simulink model "Main_C0_C3"  (R2023a)
settings: Solver=ode15s  StartTime=0.0  StopTime=1  RelTol=1e-3
model workspace (MAT data in the model file):
  C_IVD = 0.05
  E_IVD1 = 2.1
  E_IVD2 = 2.2
  E_IVD3 = 1.1
  E_IVD4 = 1.7
  E_IVD5 = 3.2
  IVD1 : object (value not decoded)
  IVD2 : object (value not decoded)
  IVD3 : object (value not decoded)
  IVD4 : object (value not decoded)
  IVD5 : object (value not decoded)
  eo_color = [1 0 0]
  io_color = [0 1 0]
  longissimus_color = [1 0 1]
  multifidus_color = [0 1 1]
  muscle_radius = 1
  psoas_color = [0 0 1]
  ra_color = [1 1 0.5]
symbols that are objects in the model workspace (value not decoded): IVD1, IVD2, IVD3, IVD4, IVD5
undefined symbols (not defined in the file or in its folder): AbdFlex, E_TLFflex, IAP_activation_AbdFlex, IAP_Pa, LeftAbdominalMuscleForce, LeftBackMuscleForce, LeftTransverse1MuscleForce, LeftTransverse2MuscleForce, RightAbdominalMuscleForce, RightBackMuscleForce, RightTransverse1MuscleForce, RightTransverse2MuscleForce, TLFflex2, X, Y, Z
libraries: nesl_utility x1235, sm_lib x960, fl_lib x6, simulink_extras x2
(part 5 of 37)

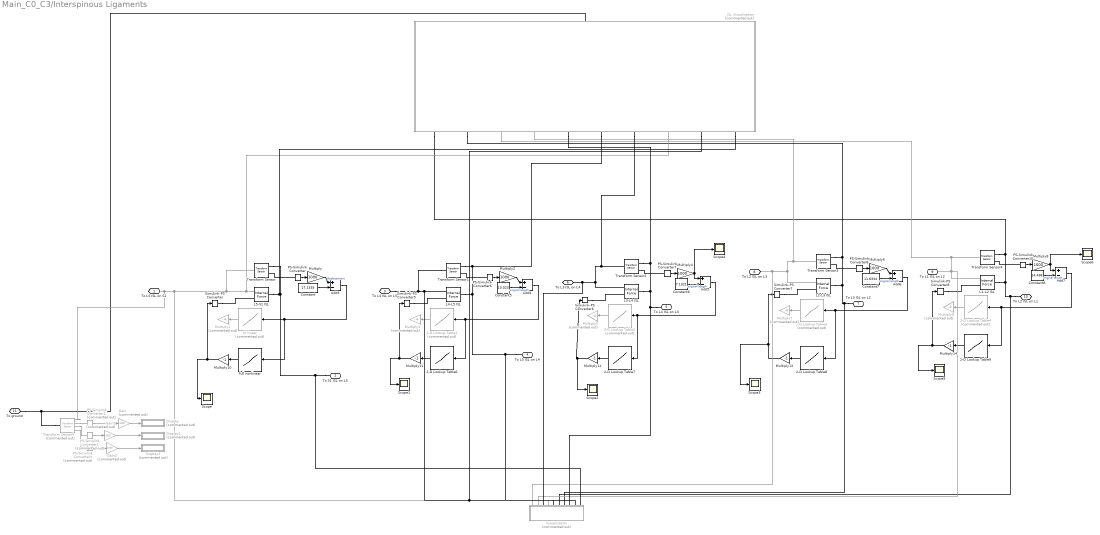
== system Main_C0_C3/Interspinous Ligaments ==
  2-D Lookup Table1 : Lookup_n-D  Commented=on  NumberOfTableDimensions=1  BreakpointsForDimension1=[0;0.1802;1.802;3.604;10.812]  BreakpointsForDimension2=[1:3]  Table=[0;0;4.82625;10.53;48.2625]  InternalRulePriority=Speed  RndMeth=Simplest
  2-D Lookup Table2 : Lookup_n-D  Commented=on  NumberOfTableDimensions=1  BreakpointsForDimension1=[0;0.054;0.54;1.08;3.24]  BreakpointsForDimension2=[1:3]  Table=[0;0;4.82625;10.53;48.2625]  InternalRulePriority=Speed  RndMeth=Simplest
  2-D Lookup Table3 : Lookup_n-D  Commented=on  NumberOfTableDimensions=1  BreakpointsForDimension1=[0;0.071;0.71;1.42;4.26]  BreakpointsForDimension2=[1:3]  Table=[0;0;4.82625;10.53;48.2625]  InternalRulePriority=Speed  RndMeth=Simplest
  2-D Lookup Table4 : Lookup_n-D  Commented=on  NumberOfTableDimensions=1  BreakpointsForDimension1=[0;0.105;1.05;2.1;6.3]  BreakpointsForDimension2=[1:3]  Table=[0;0;4.82625;10.53;48.2625]  InternalRulePriority=Speed  RndMeth=Simplest
  2-D Lookup Table6 : Lookup_n-D  NumberOfTableDimensions=1  BreakpointsForDimension1=[0;0.788999;0.899258;1.033633;1.693478;1.826126;1.958782;3.004578;3.254415;3.518032;5.870167;6.506087;7.157553]  BreakpointsForDimension2=[1:3]  Table=[0;12.24469;14.30802;16.68834;29.86456;31.92651;34.46617;57.49141;64.0048;70.67658;144.8958;168.9015;195.6133]  InternalRulePriority=Speed  RndMeth=Simplest
  2-D Lookup Table7 : Lookup_n-D  NumberOfTableDimensions=1  BreakpointsForDimension1=[0;0.432098;0.492482;0.566074;0.92744;1.000085;1.072735;1.645469;1.782294;1.926665;3.214821;3.563086;3.919864]  BreakpointsForDimension2=[1:3]  Table=[0;12.24469;14.30802;16.68834;29.86456;31.92651;34.46617;57.49141;64.0048;70.67658;144.8958;168.9015;195.6133]  InternalRulePriority=Speed  RndMeth=Simplest
  2-D Lookup Table8 : Lookup_n-D  NumberOfTableDimensions=1  BreakpointsForDimension1=[0;0.70481;0.803304;0.923341;1.512778;1.631272;1.749773;2.683979;2.907157;3.142646;5.2438;5.811865;6.393817]  BreakpointsForDimension2=[1:3]  Table=[0;12.24469;14.30802;16.68834;29.86456;31.92651;34.46617;57.49141;64.0048;70.67658;144.8958;168.9015;195.6133]  InternalRulePriority=Speed  RndMeth=Simplest
  2-D Lookup Table9 : Lookup_n-D  NumberOfTableDimensions=1  BreakpointsForDimension1=[0;0.581192;0.662411;0.761395;1.247449;1.34516;1.442878;2.213232;2.397266;2.591452;4.324082;4.792513;5.272396]  BreakpointsForDimension2=[1:3]  Table=[0;12.24469;14.30802;16.68834;29.86456;31.92651;34.46617;57.49141;64.0048;70.67658;144.8958;168.9015;195.6133]  InternalRulePriority=Speed  RndMeth=Simplest
  Add{3..7} (5 alike) : Sum  Inputs=+-
  Constant : Constant  Value=17.1335
  Constant5 : Constant  Value=13.023
  Constant6 : Constant  Value=7.1321
  Constant7 : Constant  Value=11.6334
  Constant8 : Constant  Value=14.438
  Display : Display  Commented=on
  Display1 : Display  Commented=on
  Display2 : Display  Commented=on
  Gain : Gain  Commented=on  Gain=1000
  Gain1 : Gain  Commented=on  Gain=1000
  Gain2 : Gain  Commented=on  Gain=1000
  ISL Visualization : Subsystem  Commented=on
  L1-L2 ISL : sm_lib/Forces and Torques/Internal Force
  L2-L3 ISL : sm_lib/Forces and Torques/Internal Force
  L3-L4 ISL : sm_lib/Forces and Torques/Internal Force
  L4-L5 ISL : sm_lib/Forces and Torques/Internal Force
  L5-S1 ISL : sm_lib/Forces and Torques/Internal Force
  Multiply{,2,4,6,8} (5 alike) : Gain  Gain=1000
  Multiply{1,3,5,7,9} (5 alike) : Gain  Commented=on  Gain=-4
  Multiply{10..14} (5 alike) : Gain  Gain=-1
  PS-Simulink Converter{,6..8,10} (5 alike) : nesl_utility/PS-Simulink Converter  PhysicalDomain=network_engine_domain  SubClassName=ps_output  LeftPortType=input  RightPortType=output  PseudoPeriodic=off  Frequencies=[]  VectorFormat=inherit  Unit=inherit  AffineConversion=off
  PS-Simulink Converter1 : nesl_utility/PS-Simulink Converter  Commented=on  PhysicalDomain=network_engine_domain  SubClassName=ps_output  LeftPortType=input  RightPortType=output  PseudoPeriodic=off  Frequencies=[]  VectorFormat=inherit  Unit=inherit  AffineConversion=off
  PS-Simulink Converter2 : nesl_utility/PS-Simulink Converter  Commented=on  PhysicalDomain=network_engine_domain  SubClassName=ps_output  LeftPortType=input  RightPortType=output  PseudoPeriodic=off  Frequencies=[]  VectorFormat=inherit  Unit=inherit  AffineConversion=off
  PS-Simulink Converter3 : nesl_utility/PS-Simulink Converter  Commented=on  PhysicalDomain=network_engine_domain  SubClassName=ps_output  LeftPortType=input  RightPortType=output  PseudoPeriodic=off  Frequencies=[]  VectorFormat=inherit  Unit=inherit  AffineConversion=off
  Scope{,1..6} (7 alike) : Scope
  Simulink-PS Converter{,5..8} (5 alike) : nesl_utility/Simulink-PS Converter  PhysicalDomain=network_engine_domain  SubClassName=ps_input  LeftPortType=input  RightPortType=output  PseudoPeriodic=off  Frequencies=[]  NoiseDistribution=none  NoiseParameters=[]  Unit=1  AffineConversion=off  FilteringAndDerivatives=provide  SimscapeFilterOrder=1  InputFilterTimeConstant=0.001  UdotUserProvided=0
  Transform Sensor{,1..4} (5 alike) : sm_lib/Frames and Transforms/Transform Sensor  MeasurementFrame=World  RotationSequence=XYX  SenseAngle=off  SenseAxis=off  SenseQ=off  SenseR=off  SenseRotationSequence=off  SenseOmegaX=off  SenseOmegaY=off  SenseOmegaZ=off  SenseQDot=off  SenseRDot=off  SenseRotationSequenceDot=off  SenseAlphaX=off  SenseAlphaY=off  SenseAlphaZ=off  SenseQDDot=off  SenseRDDot=off  SenseX=off  SenseY=off  SenseZ=off  SenseRad=off  SenseAzim=off  SenseDist=on  SenseInc=off  SenseXDot=off  SenseYDot=off  SenseZDot=off  SenseRadDot=off  SenseAzimDot=off  SenseDistDot=off  SenseIncDot=off  SenseXDDot=off  SenseYDDot=off  SenseZDDot=off  SenseRadDDot=off  SenseAzimDDot=off  SenseDistDDot=off  SenseIncDDot=off
  Transform Sensor5 : sm_lib/Frames and Transforms/Transform Sensor  Commented=on  MeasurementFrame=World  RotationSequence=XYZ  SenseAngle=off  SenseAxis=off  SenseQ=off  SenseR=off  SenseRotationSequence=off  SenseOmegaX=off  SenseOmegaY=off  SenseOmegaZ=off  SenseQDot=off  SenseRDot=off  SenseRotationSequenceDot=off  SenseAlphaX=off  SenseAlphaY=off  SenseAlphaZ=off  SenseQDDot=off  SenseRDDot=off  SenseX=on  SenseY=on  SenseZ=on  SenseRad=off  SenseAzim=off  SenseDist=off  SenseInc=off  SenseXDot=off  SenseYDot=off  SenseZDot=off  SenseRadDot=off  SenseAzimDot=off  SenseDistDot=off  SenseIncDot=off  SenseXDDot=off  SenseYDDot=off  SenseZDDot=off  SenseRadDDot=off  SenseAzimDDot=off  SenseDistDDot=off  SenseIncDDot=off
  Visualization : Subsystem  Commented=on
  bi linear : Lookup_n-D  Commented=on  NumberOfTableDimensions=1  BreakpointsForDimension1=[0;0.1802;1.802;3.604;10.812]  BreakpointsForDimension2=[1:3]  Table=[0;0;4.82625;10.53;48.2625]  InternalRulePriority=Speed  RndMeth=Simplest
  full nonlinear : Lookup_n-D  NumberOfTableDimensions=1  BreakpointsForDimension1=[0;1.038033;1.183094;1.359883;2.227997;2.402513;2.57704;3.952924;4.281618;4.628442;7.722991;8.559628;9.41672]  BreakpointsForDimension2=[1:3]  Table=[0;12.24469;14.30802;16.68834;29.86456;31.92651;34.46617;57.49141;64.0048;70.67658;144.8958;168.9015;195.6133]  InternalRulePriority=Speed  RndMeth=Simplest
  To L5 ISL on S1 : PMIOPort  Side=Left
  To S1 ISL on L5 : PMIOPort  Port=2  Side=Left
  To L4 ISL on L5 : PMIOPort  Port=3  Side=Left
  To L5 ISL on L4 : PMIOPort  Port=4  Side=Left
  To L4 ISL on L3 : PMIOPort  Port=5  Side=Left
  To L3 ISL on L4 : PMIOPort  Port=6  Side=Left
  To L3 ISL on L2 : PMIOPort  Port=7  Side=Left
  To L2 ISL on L3 : PMIOPort  Port=8  Side=Left
  To L1 ISL on L2 : PMIOPort  Port=9  Side=Left
  To L2 ISL on L1 : PMIOPort  Port=10  Side=Left
  "To ground " : PMIOPort  Port=11  Side=Left
  wires:
  Multiply10/1 -> Simulink-PS Converter/1, Scope/1
  Gain/1 -> Display/1
  Gain1/1 -> Display1/1
  Gain2/1 -> Display2/1
  PS-Simulink Converter3/1 -> Gain2/1
  PS-Simulink Converter2/1 -> Gain1/1
  PS-Simulink Converter1/1 -> Gain/1
  Multiply14/1 -> Scope5/1, Simulink-PS Converter8/1
  Multiply13/1 -> Simulink-PS Converter7/1, Scope3/1
  Multiply12/1 -> Simulink-PS Converter6/1, Scope2/1
  Multiply11/1 -> Simulink-PS Converter5/1, Scope1/1
  2-D Lookup Table9/1 -> Multiply14/1
  2-D Lookup Table8/1 -> Multiply13/1
  2-D Lookup Table7/1 -> Multiply12/1
  2-D Lookup Table6/1 -> Multiply11/1
  full nonlinear/1 -> Multiply10/1
  Add7/1 -> 2-D Lookup Table4/1, 2-D Lookup Table9/1
  Constant8/1 -> Add7/2  "original length"
  Constant7/1 -> Add6/2  "original length"
  Add6/1 -> 2-D Lookup Table3/1, 2-D Lookup Table8/1
  Add5/1 -> 2-D Lookup Table2/1, 2-D Lookup Table7/1
  Constant6/1 -> Add5/2  "original length"
  Constant5/1 -> Add4/2  "original length"
  Add4/1 -> 2-D Lookup Table1/1, 2-D Lookup Table6/1
  Multiply/1 -> Add3/1  "displacement"
  PS-Simulink Converter10/1 -> Multiply8/1
  PS-Simulink Converter8/1 -> Multiply6/1
  Multiply6/1 -> Add6/1
  PS-Simulink Converter/1 -> Multiply/1
  bi linear/1 -> Multiply1/1
  2-D Lookup Table4/1 -> Multiply9/1
  Constant/1 -> Add3/2
  PS-Simulink Converter7/1 -> Multiply4/1
  2-D Lookup Table3/1 -> Multiply7/1
  2-D Lookup Table2/1 -> Multiply5/1
  PS-Simulink Converter6/1 -> Multiply2/1
  Multiply2/1 -> Add4/1
  2-D Lookup Table1/1 -> Multiply3/1
  Multiply4/1 -> Scope4/1, Add5/1
  Add3/1 -> bi linear/1, full nonlinear/1
  Multiply8/1 -> Scope6/1, Add7/1
  connections:
  Transform Sensor5/LConn1 -- ISL Visualization/LConn1 -- "To ground "/RConn1
  Transform Sensor5/RConn4 -- PS-Simulink Converter3/LConn1
  Transform Sensor5/RConn3 -- PS-Simulink Converter2/LConn1
  Transform Sensor5/RConn2 -- PS-Simulink Converter1/LConn1
  To L2 ISL on L1/RConn1 -- Visualization/LConn6 -- Transform Sensor4/RConn1 -- ISL Visualization/RConn1 -- L1-L2 ISL/RConn1
  ISL Visualization/RConn4 -- Transform Sensor3/LConn1 -- To L2 ISL on L3/RConn1 -- Visualization/LConn1 -- L2-L3 ISL/LConn1
  Simulink-PS Converter7/RConn1 -- L2-L3 ISL/LConn2
  PS-Simulink Converter10/LConn1 -- Transform Sensor4/RConn2
  PS-Simulink Converter7/LConn1 -- Transform Sensor2/RConn2
  Simulink-PS Converter8/RConn1 -- L1-L2 ISL/LConn2
  PS-Simulink Converter/LConn1 -- Transform Sensor/RConn2
  Simulink-PS Converter6/RConn1 -- L3-L4 ISL/LConn2
  To L3 ISL on L2/RConn1 -- Visualization/LConn7 -- ISL Visualization/RConn2 -- Transform Sensor3/RConn1 -- L2-L3 ISL/RConn1
  ISL Visualization/RConn8 -- To L5 ISL on S1/RConn1 -- Transform Sensor5/RConn1 -- Visualization/LConn4 -- Transform Sensor/LConn1 -- L5-S1 ISL/LConn1
  Simulink-PS Converter5/RConn1 -- L4-L5 ISL/LConn2
  ISL Visualization/RConn3 -- Transform Sensor4/LConn1 -- Visualization/LConn2 -- To L1 ISL on L2/RConn1 -- L1-L2 ISL/LConn1
  To L3 ISL on L4/RConn1 -- Visualization/LConn3 -- Transform Sensor2/LConn1 -- ISL Visualization/RConn7 -- L3-L4 ISL/LConn1
  To S1 ISL on L5/RConn1 -- Visualization/LConn10 -- Transform Sensor/RConn1 -- ISL Visualization/RConn10 -- L5-S1 ISL/RConn1
  To L4 ISL on L3/RConn1 -- Visualization/LConn8 -- Transform Sensor2/RConn1 -- ISL Visualization/RConn5 -- L3-L4 ISL/RConn1
  To L5 ISL on L4/RConn1 -- Visualization/LConn9 -- ISL Visualization/RConn6 -- Transform Sensor1/RConn1 -- L4-L5 ISL/RConn1
  PS-Simulink Converter8/LConn1 -- Transform Sensor3/RConn2
  Transform Sensor1/LConn1 -- To L4 ISL on L5/RConn1 -- ISL Visualization/RConn9 -- Visualization/LConn5 -- L4-L5 ISL/LConn1
  PS-Simulink Converter6/LConn1 -- Transform Sensor1/RConn2
  Simulink-PS Converter/RConn1 -- L5-S1 ISL/LConn2

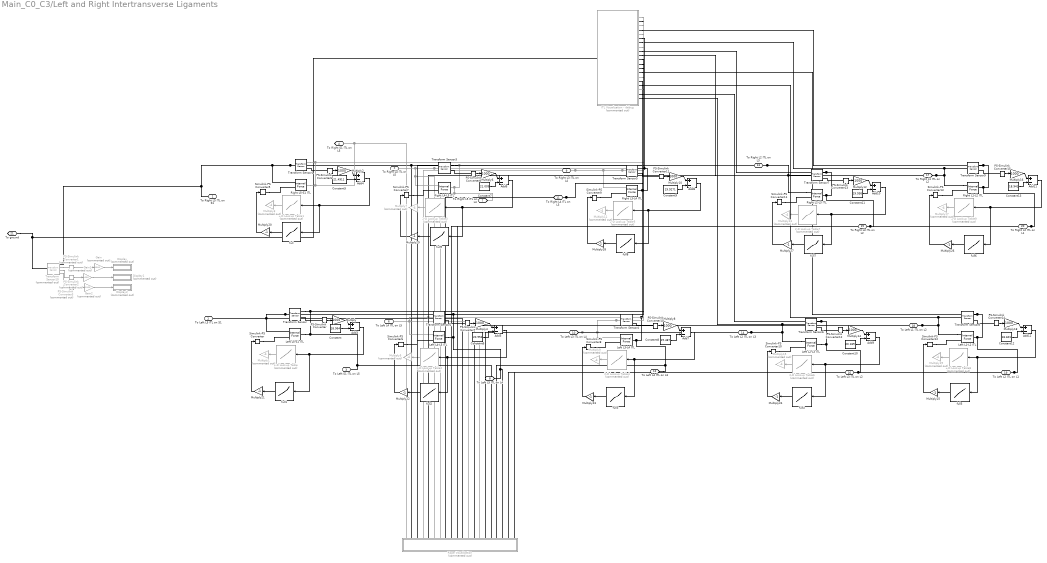
== system Main_C0_C3/Left and Right Intertransverse Ligaments ==
  2-D Lookup Table : Lookup_n-D  Commented=on  NumberOfTableDimensions=1  BreakpointsForDimension1=[0;0.178;2.67;3.916;5.34]  BreakpointsForDimension2=[1:3]  Table=[0;0;3;7.5;30]  InternalRulePriority=Speed  RndMeth=Simplest
  2-D Lookup Table1 : Lookup_n-D  Commented=on  NumberOfTableDimensions=1  BreakpointsForDimension1=[0;0.178;2.67;3.916;5.34]  BreakpointsForDimension2=[1:3]  Table=[0;0;3;7.5;30]  InternalRulePriority=Speed  RndMeth=Simplest
  2-D Lookup Table2 : Lookup_n-D  Commented=on  NumberOfTableDimensions=1  BreakpointsForDimension1=[0;0.213;3.195;4.686;6.39]  BreakpointsForDimension2=[1:3]  Table=[0;0;3;7.5;30]  InternalRulePriority=Speed  RndMeth=Simplest
  2-D Lookup Table3 : Lookup_n-D  Commented=on  NumberOfTableDimensions=1  BreakpointsForDimension1=[0;0.213;3.195;4.686;6.39]  BreakpointsForDimension2=[1:3]  Table=[0;0;3;7.5;30]  InternalRulePriority=Speed  RndMeth=Simplest
  2-D Lookup Table4 : Lookup_n-D  Commented=on  NumberOfTableDimensions=1  BreakpointsForDimension1=[0;0.1985;2.9775;4.367;5.955]  BreakpointsForDimension2=[1:3]  Table=[0;0;3;7.5;30]  InternalRulePriority=Speed  RndMeth=Simplest
  2-D Lookup Table5 : Lookup_n-D  Commented=on  NumberOfTableDimensions=1  BreakpointsForDimension1=[0;0.1985;2.9775;4.367;5.955]  BreakpointsForDimension2=[1:3]  Table=[0;0;3;7.5;30]  InternalRulePriority=Speed  RndMeth=Simplest
  2-D Lookup Table6 : Lookup_n-D  Commented=on  NumberOfTableDimensions=1  BreakpointsForDimension1=[0;0.2084;3.126;4.5848;6.252]  BreakpointsForDimension2=[1:3]  Table=[0;0;3;7.5;30]  InternalRulePriority=Speed  RndMeth=Simplest
  2-D Lookup Table7 : Lookup_n-D  Commented=on  NumberOfTableDimensions=1  BreakpointsForDimension1=[0;0.2084;3.126;4.5848;6.252]  BreakpointsForDimension2=[1:3]  Table=[0;0;3;7.5;30]  InternalRulePriority=Speed  RndMeth=Simplest
  2-D Lookup Table8 : Lookup_n-D  Commented=on  NumberOfTableDimensions=1  BreakpointsForDimension1=[0;0.1966;2.949;4.3252;5.898]  BreakpointsForDimension2=[1:3]  Table=[0;0;3;7.5;30]  InternalRulePriority=Speed  RndMeth=Simplest
  2-D Lookup Table9 : Lookup_n-D  Commented=on  NumberOfTableDimensions=1  BreakpointsForDimension1=[0;0.1966;2.949;4.3252;5.898]  BreakpointsForDimension2=[1:3]  Table=[0;0;3;7.5;30]  InternalRulePriority=Speed  RndMeth=Simplest
  Add{3..12} (10 alike) : Sum  Inputs=+-
  Constant : Constant  Value=18.964
  Constant10 : Constant  Value=20.189
  Constant11 : Constant  Value=19.936
  Constant12 : Constant  Value=18.601
  Constant13 : Constant  Value=18.941
  Constant5 : Constant  Value=21.4911
  Constant6 : Constant  Value=20.952
  Constant7 : Constant  Value=21.009
  Constant8 : Constant  Value=19.487
  Constant9 : Constant  Value=19.9271
  Display : Display  Commented=on
  Display1 : Display  Commented=on
  Display2 : Display  Commented=on
  Gain : Gain  Commented=on  Gain=1000
  Gain1 : Gain  Commented=on  Gain=1000
  Gain2 : Gain  Commented=on  Gain=1000
  ITL Visualization - debug : Subsystem  Commented=on
  Left L1-L2 ITL : sm_lib/Forces and Torques/Internal Force
  Left L2-L3 ITL : sm_lib/Forces and Torques/Internal Force
  Left L3-L4 ITL : sm_lib/Forces and Torques/Internal Force
  Left L4-L5 ITL : sm_lib/Forces and Torques/Internal Force
  Left L5-S1 ITL : sm_lib/Forces and Torques/Internal Force
  Multiply{,2,4,6,8,10,12,14,16,18} (10 alike) : Gain  Gain=1000
  Multiply{1,3,5,7,9,11,13,15,17,19} (10 alike) : Gain  Commented=on  Gain=-4
  Multiply{20..29} (10 alike) : Gain  Gain=-1
  PS-Simulink Converter{,6..8,10..15} (10 alike) : nesl_utility/PS-Simulink Converter  PhysicalDomain=network_engine_domain  SubClassName=ps_output  LeftPortType=input  RightPortType=output  PseudoPeriodic=off  Frequencies=[]  VectorFormat=inherit  Unit=inherit  AffineConversion=off
  PS-Simulink Converter1 : nesl_utility/PS-Simulink Converter  Commented=on  PhysicalDomain=network_engine_domain  SubClassName=ps_output  LeftPortType=input  RightPortType=output  PseudoPeriodic=off  Frequencies=[]  VectorFormat=inherit  Unit=inherit  AffineConversion=off
  PS-Simulink Converter2 : nesl_utility/PS-Simulink Converter  Commented=on  PhysicalDomain=network_engine_domain  SubClassName=ps_output  LeftPortType=input  RightPortType=output  PseudoPeriodic=off  Frequencies=[]  VectorFormat=inherit  Unit=inherit  AffineConversion=off
  PS-Simulink Converter3 : nesl_utility/PS-Simulink Converter  Commented=on  PhysicalDomain=network_engine_domain  SubClassName=ps_output  LeftPortType=input  RightPortType=output  PseudoPeriodic=off  Frequencies=[]  VectorFormat=inherit  Unit=inherit  AffineConversion=off
  Right L1-L2 ITL : sm_lib/Forces and Torques/Internal Force
  Right L2-L3 ITL : sm_lib/Forces and Torques/Internal Force
  Right L3-L4 ITL : sm_lib/Forces and Torques/Internal Force
  Right L4-L5 ITL : sm_lib/Forces and Torques/Internal Force
  Right L5-S1 ITL : sm_lib/Forces and Torques/Internal Force
  Rope Visualization : Subsystem  Commented=on
  Simulink-PS Converter{,5..13} (10 alike) : nesl_utility/Simulink-PS Converter  PhysicalDomain=network_engine_domain  SubClassName=ps_input  LeftPortType=input  RightPortType=output  PseudoPeriodic=off  Frequencies=[]  NoiseDistribution=none  NoiseParameters=[]  Unit=1  AffineConversion=off  FilteringAndDerivatives=provide  SimscapeFilterOrder=1  InputFilterTimeConstant=0.001  UdotUserProvided=0
  Transform Sensor{,1..9} (10 alike) : sm_lib/Frames and Transforms/Transform Sensor  MeasurementFrame=World  RotationSequence=XYX  SenseAngle=off  SenseAxis=off  SenseQ=off  SenseR=off  SenseRotationSequence=off  SenseOmegaX=off  SenseOmegaY=off  SenseOmegaZ=off  SenseQDot=off  SenseRDot=off  SenseRotationSequenceDot=off  SenseAlphaX=off  SenseAlphaY=off  SenseAlphaZ=off  SenseQDDot=off  SenseRDDot=off  SenseX=off  SenseY=off  SenseZ=off  SenseRad=off  SenseAzim=off  SenseDist=on  SenseInc=off  SenseXDot=off  SenseYDot=off  SenseZDot=off  SenseRadDot=off  SenseAzimDot=off  SenseDistDot=off  SenseIncDot=off  SenseXDDot=off  SenseYDDot=off  SenseZDDot=off  SenseRadDDot=off  SenseAzimDDot=off  SenseDistDDot=off  SenseIncDDot=off
  Transform Sensor10 : sm_lib/Frames and Transforms/Transform Sensor  Commented=on  MeasurementFrame=World  RotationSequence=XYZ  SenseAngle=off  SenseAxis=off  SenseQ=off  SenseR=off  SenseRotationSequence=off  SenseOmegaX=off  SenseOmegaY=off  SenseOmegaZ=off  SenseQDot=off  SenseRDot=off  SenseRotationSequenceDot=off  SenseAlphaX=off  SenseAlphaY=off  SenseAlphaZ=off  SenseQDDot=off  SenseRDDot=off  SenseX=on  SenseY=on  SenseZ=on  SenseRad=off  SenseAzim=off  SenseDist=off  SenseInc=off  SenseXDot=off  SenseYDot=off  SenseZDot=off  SenseRadDot=off  SenseAzimDot=off  SenseDistDot=off  SenseIncDot=off  SenseXDDot=off  SenseYDDot=off  SenseZDDot=off  SenseRadDDot=off  SenseAzimDDot=off  SenseDistDDot=off  SenseIncDDot=off
  full : Lookup_n-D  NumberOfTableDimensions=1  BreakpointsForDimension1=[0;3.246412;4.726972;5.305443;5.825602;6.352653]  BreakpointsForDimension2=[1:3]  Table=[0;12.07558;29.7358;59.62187;90.36674;120.0008]  InternalRulePriority=Speed  RndMeth=Simplest
  full1 : Lookup_n-D  NumberOfTableDimensions=1  BreakpointsForDimension1=[0;2.864673;4.171136;4.681585;5.14058;5.605656]  BreakpointsForDimension2=[1:3]  Table=[0;12.07558;29.7358;59.62187;90.36674;120.0008]  InternalRulePriority=Speed  RndMeth=Simplest
  full2 : Lookup_n-D  NumberOfTableDimensions=1  BreakpointsForDimension1=[0;3.164977;4.608397;5.172357;5.679468;6.193298]  BreakpointsForDimension2=[1:3]  Table=[0;12.07558;29.7358;59.62187;90.36674;120.0008]  InternalRulePriority=Speed  RndMeth=Simplest
  full3 : Lookup_n-D  NumberOfTableDimensions=1  BreakpointsForDimension1=[0;2.943676;4.28617;4.810697;5.28235;5.760252]  BreakpointsForDimension2=[1:3]  Table=[0;12.07558;29.7358;59.62187;90.36674;120.0008]  InternalRulePriority=Speed  RndMeth=Simplest
  full4 : Lookup_n-D  NumberOfTableDimensions=1  BreakpointsForDimension1=[0;3.049719;4.440575;4.983997;5.472641;5.967759]  BreakpointsForDimension2=[1:3]  Table=[0;12.07558;29.7358;59.62187;90.36674;120.0008]  InternalRulePriority=Speed  RndMeth=Simplest
  full5 : Lookup_n-D  NumberOfTableDimensions=1  BreakpointsForDimension1=[0;2.809838;4.091294;4.591973;5.042181;5.498355]  BreakpointsForDimension2=[1:3]  Table=[0;12.07558;29.7358;59.62187;90.36674;120.0008]  InternalRulePriority=Speed  RndMeth=Simplest
  full6 : Lookup_n-D  NumberOfTableDimensions=1  BreakpointsForDimension1=[0;2.861198;4.166077;4.675907;5.134345;5.598857]  BreakpointsForDimension2=[1:3]  Table=[0;12.07558;29.7358;59.62187;90.36674;120.0008]  InternalRulePriority=Speed  RndMeth=Simplest
  full7 : Lookup_n-D  NumberOfTableDimensions=1  BreakpointsForDimension1=[0;3.011501;4.384927;4.92154;5.40406;5.892974]  BreakpointsForDimension2=[1:3]  Table=[0;12.07558;29.7358;59.62187;90.36674;120.0008]  InternalRulePriority=Speed  RndMeth=Simplest
  full8 : Lookup_n-D  NumberOfTableDimensions=1  BreakpointsForDimension1=[0;3.010157;4.38297;4.919343;5.401648;5.890343]  BreakpointsForDimension2=[1:3]  Table=[0;12.07558;29.7358;59.62187;90.36674;120.0008]  InternalRulePriority=Speed  RndMeth=Simplest
  full9 : Lookup_n-D  NumberOfTableDimensions=1  BreakpointsForDimension1=[0;3.173587;4.620934;5.186428;5.694919;6.210147]  BreakpointsForDimension2=[1:3]  Table=[0;12.07558;29.7358;59.62187;90.36674;120.0008]  InternalRulePriority=Speed  RndMeth=Simplest
  To Right L5 ITL on S1 : PMIOPort  Side=Left
  To Left L5 ITL on S1 : PMIOPort  Port=2  Side=Left
  To Left S1 ITL on L5 : PMIOPort  Port=3  Side=Left
  To Right S1 ITL on L5 : PMIOPort  Port=4  Side=Left
  To Right L4 ITL on L5 : PMIOPort  Port=5  Side=Left
  To Left L4 ITL on L5 : PMIOPort  Port=6  Side=Left
  To Right L5 ITL on L4 : PMIOPort  Port=7  Side=Left
  To Left L5 ITL on L4 : PMIOPort  Port=8  Side=Left
  To Right L3 ITL on L4 : PMIOPort  Port=9  Side=Left
  To Left L3 ITL on L4 : PMIOPort  Port=10  Side=Left
  To Right L4 ITL on L3 : PMIOPort  Port=11  Side=Left
  To Left L4 ITL on L3 : PMIOPort  Port=12  Side=Left
  To Right L2 ITL on L3 : PMIOPort  Port=13  Side=Left
  To Left L2 ITL on L3 : PMIOPort  Port=14  Side=Left
  To Right L3 ITL on L2 : PMIOPort  Port=15  Side=Left
  To Left L3 ITL on L2 : PMIOPort  Port=16  Side=Left
  To Right L1 ITL on L2 : PMIOPort  Port=17  Side=Left
  To Left L1 ITL on L2 : PMIOPort  Port=18  Side=Left
  To Left L2 ITL on L1 : PMIOPort  Port=19  Side=Left
  To Right L2 ITL on L1 : PMIOPort  Port=20  Side=Left
  To ground : PMIOPort  Port=21  Side=Left
  wires:
  Gain2/1 -> Display2/1
  Gain1/1 -> Display1/1
  PS-Simulink Converter1/1 -> Gain/1
  PS-Simulink Converter2/1 -> Gain1/1
  PS-Simulink Converter3/1 -> Gain2/1
  Gain/1 -> Display/1
  Multiply22/1 -> Simulink-PS Converter6/1
  Multiply23/1 -> Simulink-PS Converter8/1
  Multiply24/1 -> Simulink-PS Converter10/1
  Multiply25/1 -> Simulink-PS Converter12/1
  Multiply26/1 -> Simulink-PS Converter13/1
  Multiply27/1 -> Simulink-PS Converter11/1
  Multiply28/1 -> Simulink-PS Converter9/1
  Multiply29/1 -> Simulink-PS Converter7/1
  Multiply21/1 -> Simulink-PS Converter/1
  full9/1 -> Multiply29/1
  full8/1 -> Multiply28/1
  full7/1 -> Multiply27/1
  full6/1 -> Multiply26/1
  full5/1 -> Multiply25/1
  full4/1 -> Multiply24/1
  full3/1 -> Multiply23/1
  full2/1 -> Multiply22/1
  full1/1 -> Multiply21/1
  Multiply20/1 -> Simulink-PS Converter5/1
  full/1 -> Multiply20/1
  PS-Simulink Converter6/1 -> Multiply2/1
  Multiply2/1 -> Add4/1
  2-D Lookup Table1/1 -> Multiply3/1
  Add4/1 -> 2-D Lookup Table1/1, full/1
  Constant5/1 -> Add4/2
  Multiply12/1 -> Add10/1
  PS-Simulink Converter13/1 -> Multiply12/1
  PS-Simulink Converter/1 -> Multiply/1
  Add3/1 -> 2-D Lookup Table/1, full1/1
  2-D Lookup Table7/1 -> Multiply13/1
  Multiply/1 -> Add3/1
  Constant/1 -> Add3/2
  2-D Lookup Table6/1 -> Multiply15/1
  Add10/1 -> 2-D Lookup Table7/1, full7/1
  Constant10/1 -> Add9/2
  Add9/1 -> 2-D Lookup Table6/1, full4/1
  PS-Simulink Converter12/1 -> Multiply14/1
  2-D Lookup Table5/1 -> Multiply11/1
  Multiply10/1 -> Add8/1
  PS-Simulink Converter11/1 -> Multiply10/1
  2-D Lookup Table4/1 -> Multiply9/1
  PS-Simulink Converter14/1 -> Multiply18/1
  PS-Simulink Converter10/1 -> Multiply8/1
  Constant13/1 -> Add11/2
  Add11/1 -> 2-D Lookup Table9/1, full6/1
  PS-Simulink Converter15/1 -> Multiply16/1
  Add7/1 -> 2-D Lookup Table4/1, full3/1
  Multiply4/1 -> Add5/1
  2-D Lookup Table2/1 -> Multiply5/1
  Multiply8/1 -> Add7/1
  Multiply14/1 -> Add9/1
  Constant7/1 -> Add6/2
  Constant8/1 -> Add7/2
  Constant12/1 -> Add12/2
  PS-Simulink Converter7/1 -> Multiply4/1
  Multiply6/1 -> Add6/1
  PS-Simulink Converter8/1 -> Multiply6/1
  2-D Lookup Table3/1 -> Multiply7/1
  2-D Lookup Table8/1 -> Multiply19/1
  2-D Lookup Table9/1 -> Multiply17/1
  Constant11/1 -> Add10/2
  Add6/1 -> 2-D Lookup Table3/1, full9/1
  2-D Lookup Table/1 -> Multiply1/1
  Multiply16/1 -> Add11/1
  Add5/1 -> 2-D Lookup Table2/1, full2/1
  Constant9/1 -> Add8/2
  Constant6/1 -> Add5/2
  Add12/1 -> 2-D Lookup Table8/1, full5/1
  Add8/1 -> 2-D Lookup Table5/1, full8/1
  Multiply18/1 -> Add12/1
  connections:
  To ground/RConn1 -- ITL Visualization - debug/LConn1 -- Transform Sensor10/LConn1
  Transform Sensor10/RConn2 -- PS-Simulink Converter1/LConn1
  Transform Sensor10/RConn3 -- PS-Simulink Converter2/LConn1
  Transform Sensor10/RConn4 -- PS-Simulink Converter3/LConn1
  ITL Visualization - debug/RConn8 -- Right L3-L4 ITL/LConn1 -- To Right L3 ITL on L4/RConn1 -- Rope Visualization/LConn4 -- Transform Sensor5/LConn1
  Transform Sensor8/RConn1 -- ITL Visualization - debug/RConn14 -- To Left L2 ITL on L1/RConn1 -- Rope Visualization/LConn20 -- Left L1-L2 ITL/RConn1
  PS-Simulink Converter6/LConn1 -- Transform Sensor1/RConn2
  Right L5-S1 ITL/LConn1 -- To Right L5 ITL on S1/RConn1 -- Transform Sensor10/RConn1 -- ITL Visualization - debug/RConn2 -- Rope Visualization/LConn2 -- Transform Sensor1/LConn1
  Rope Visualization/LConn1 -- To Right S1 ITL on L5/RConn1 -- Transform Sensor1/RConn1 -- ITL Visualization - debug/RConn1 -- Right L5-S1 ITL/RConn1
  PS-Simulink Converter12/LConn1 -- Transform Sensor6/RConn2
  Simulink-PS Converter/RConn1 -- Left L5-S1 ITL/LConn2
  PS-Simulink Converter/LConn1 -- Transform Sensor/RConn2
  Transform Sensor/LConn1 -- ITL Visualization - debug/RConn12 -- To Left L5 ITL on S1/RConn1 -- Rope Visualization/LConn11 -- Left L5-S1 ITL/LConn1
  PS-Simulink Converter11/LConn1 -- Transform Sensor5/RConn2
  Simulink-PS Converter9/RConn1 -- Right L3-L4 ITL/LConn2
  PS-Simulink Converter14/LConn1 -- Transform Sensor8/RConn2
  Simulink-PS Converter13/RConn1 -- Right L1-L2 ITL/LConn2
  Transform Sensor4/RConn1 -- ITL Visualization - debug/RConn16 -- To Left L4 ITL on L3/RConn1 -- Rope Visualization/LConn17 -- Left L3-L4 ITL/RConn1
  Simulink-PS Converter5/RConn1 -- Right L5-S1 ITL/LConn2
  PS-Simulink Converter15/LConn1 -- Transform Sensor9/RConn2
  Rope Visualization/LConn7 -- To Right L5 ITL on L4/RConn1 -- Transform Sensor3/RConn1 -- ITL Visualization - debug/RConn3 -- Right L4-L5 ITL/RConn1
  PS-Simulink Converter10/LConn1 -- Transform Sensor4/RConn2
  ITL Visualization - debug/RConn15 -- Left L4-L5 ITL/LConn1 -- Rope Visualization/LConn12 -- To Left L4 ITL on L5/RConn1 -- Transform Sensor2/LConn1
  Right L1-L2 ITL/LConn1 -- To Right L1 ITL on L2/RConn1 -- Rope Visualization/LConn5 -- ITL Visualization - debug/RConn7 -- Transform Sensor9/LConn1
  PS-Simulink Converter8/LConn1 -- Transform Sensor3/RConn2
  ITL Visualization - debug/RConn5 -- To Right L4 ITL on L5/RConn1 -- Right L4-L5 ITL/LConn1 -- Rope Visualization/LConn6 -- Transform Sensor3/LConn1
  PS-Simulink Converter7/LConn1 -- Transform Sensor2/RConn2
  Simulink-PS Converter8/RConn1 -- Left L3-L4 ITL/LConn2
  ITL Visualization - debug/RConn18 -- Left L3-L4 ITL/LConn1 -- To Left L3 ITL on L4/RConn1 -- Rope Visualization/LConn14 -- Transform Sensor4/LConn1
  Left L1-L2 ITL/LConn1 -- To Left L1 ITL on L2/RConn1 -- Rope Visualization/LConn13 -- ITL Visualization - debug/RConn17 -- Transform Sensor8/LConn1
  Simulink-PS Converter7/RConn1 -- Right L4-L5 ITL/LConn2
  To Left S1 ITL on L5/RConn1 -- Rope Visualization/LConn16 -- ITL Visualization - debug/RConn11 -- Transform Sensor/RConn1 -- Left L5-S1 ITL/RConn1
  Simulink-PS Converter10/RConn1 -- Left L2-L3 ITL/LConn2
  PS-Simulink Converter13/LConn1 -- Transform Sensor7/RConn2
  Simulink-PS Converter6/RConn1 -- Left L4-L5 ITL/LConn2
  Simulink-PS Converter11/RConn1 -- Right L2-L3 ITL/LConn2
  Transform Sensor6/RConn1 -- ITL Visualization - debug/RConn19 -- To Left L3 ITL on L2/RConn1 -- Rope Visualization/LConn19 -- Left L2-L3 ITL/RConn1
  Transform Sensor5/RConn1 -- ITL Visualization - debug/RConn6 -- To Right L4 ITL on L3/RConn1 -- Rope Visualization/LConn8 -- Right L3-L4 ITL/RConn1
  Simulink-PS Converter12/RConn1 -- Left L1-L2 ITL/LConn2
  To Left L5 ITL on L4/RConn1 -- Rope Visualization/LConn18 -- Transform Sensor2/RConn1 -- ITL Visualization - debug/RConn13 -- Left L4-L5 ITL/RConn1
  Transform Sensor9/RConn1 -- ITL Visualization - debug/RConn4 -- To Right L2 ITL on L1/RConn1 -- Rope Visualization/LConn10 -- Right L1-L2 ITL/RConn1
  Left L2-L3 ITL/LConn1 -- To Left L2 ITL on L3/RConn1 -- Rope Visualization/LConn15 -- ITL Visualization - debug/RConn20 -- Transform Sensor6/LConn1
  Right L2-L3 ITL/LConn1 -- ITL Visualization - debug/RConn10 -- To Right L2 ITL on L3/RConn1 -- Rope Visualization/LConn3 -- Transform Sensor7/LConn1
  Transform Sensor7/RConn1 -- ITL Visualization - debug/RConn9 -- To Right L3 ITL on L2/RConn1 -- Rope Visualization/LConn9 -- Right L2-L3 ITL/RConn1
